simulink model "Project_Observer_Continuous"  (R2014a)
settings: Solver=ode45  StartTime=0.0  StopTime=5  RelTol=1e-3
values from neighbouring files (symbols this model uses):
  A = [-(Kt*Kb/Ra/Je+Be/Je),0;1,0]    [Lab_6_01.m]
  B = [Kt/Ra/Je;0]    [Lab_6_01.m]
  Be = Bm    (= 0.02)    [Lab_6_01.m]
  C = [0,rm*r2/r1]    [Lab_6_01.m]
  Je = Jo+Jm+(rm/r1)^2*(J1+J2)+mc*(rm*r2/r1)^2+J3*(rm*r2/(r1*r3))^2    [Lab_6_01.m]
  K = [0,1]*(Pc^-1)*qa    [Lab_6_01.m]
  Kb = 0.060    (= 0.06)    [Lab_6_01.m]
  Kt = 0.065    [Lab_6_01.m]
  L = pa*Po^-1*[0;1]    [Lab_6_01.m]
  La = 0    [Lab_6_01.m]
  n = rm*r2/r1    (= 0.15)    [Lab_6_01.m]
  pos = input('Enter desired steady-state position [mm]: ')/1000    [Lab_6_01.m]
  Ra = 1.5    [Lab_6_01.m]
  ramp = input('Enter desired steady-state velocity [mm/s]: ')/1000    [Lab_6_01.m]
  Ramp_On = 1    [Lab_6_01.m]
  SampleTime = 0.01    [Lab_6_01.m]
  Step_On = 0    [Lab_6_01.m]
libraries: simulink x1
settings Model: Creator=muellerb  LastModifiedBy=cloughj

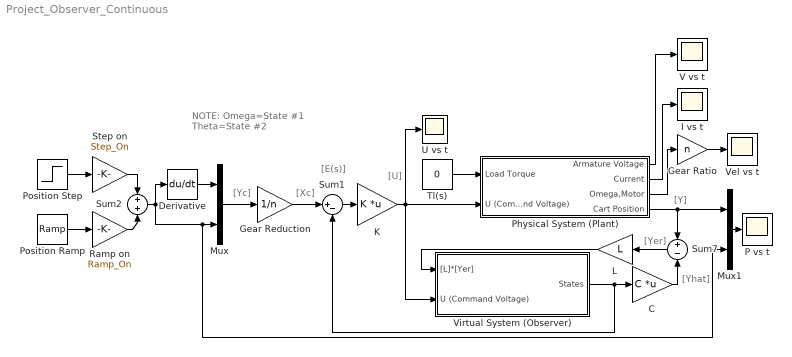
== system Project_Observer_Continuous ==
  note: [Yhat]
  note: [Yer]
  note: [Y]
  note: [U]
  note: [E(s)]
  note: [Xc]
  note: [Yc]
  note: NOTE:
      | Omega=State #1
      | Theta=State #2
  C : Gain  Gain=C  Multiplication=Matrix(K*u)
  Derivative : Derivative
  Gear Ratio : Gain  Gain=n
  Gear Reduction : Gain  Gain=1/n
  I vs t : Scope
      settings: SaveName=Current
  K : Gain  Gain=K  Multiplication=Matrix(K*u)
  L : Gain  Gain=L
  Mux : Mux  Inputs=2
  Mux1 : Mux  Inputs=2
  P vs t : Scope
      settings: SaveName=Position
  Physical System (Plant) : Subsystem
  Position Ramp : simulink/Sources/Ramp  slope=ramp  start=0  X0=0
  Position Step : Step  Time=0  After=pos  SampleTime=SampleTime
  Ramp on : Gain  Gain=Ramp_On
  Step on : Gain  Gain=Step_On
  Sum1 : Sum  Inputs=|+-
  Sum2 : Sum  Inputs=+|+
  Sum7 : Sum  Inputs=+|-
  Tl(s) : Constant  Value=0
  U vs t : Scope
      settings: SaveName=ScopeData4
  V vs t : Scope
      settings: SaveName=Voltage
  Vel vs t : Scope
      settings: SaveName=ScopeData3
  Virtual System (Observer) : Subsystem
  wires:
  Gear Ratio/1 -> Vel vs t/1
  Sum7/1 -> L/1
  Mux/1 -> Gear Reduction/1
  Gear Reduction/1 -> Sum1/1
  Sum1/1 -> K/1
  Tl(s)/1 -> Physical System (Plant)/1(Load Torque)
  Physical System (Plant)/1(Armature Voltage) -> V vs t/1
  Physical System (Plant)/2(Current) -> I vs t/1
  Physical System (Plant)/3(Omega,Motor) -> Gear Ratio/1
  Physical System (Plant)/4(Cart Position) -> Sum7/1, Mux1/1
  L/1 -> Virtual System (Observer)/1("[L]*[Yer]")
  C/1 -> Sum7/2
  Virtual System (Observer)/1(States) -> Sum1/2, C/1
  Position Ramp/1 -> Ramp on/1
  Position Step/1 -> Step on/1
  Step on/1 -> Sum2/1
  Ramp on/1 -> Sum2/2
  K/1 -> U vs t/1, Virtual System (Observer)/2(U (Command Voltage)), Physical System (Plant)/2(U (Command Voltage))
  Derivative/1 -> Mux/1
  Sum2/1 -> Mux1/2, Mux/2, Derivative/1
  Mux1/1 -> P vs t/1

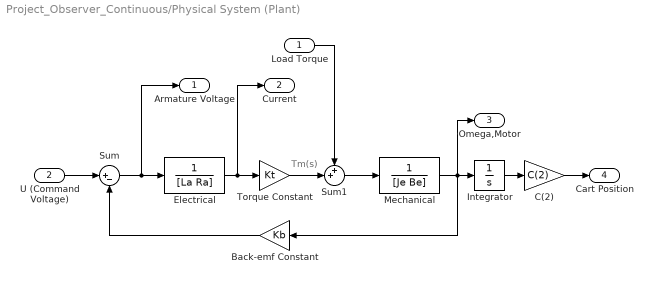
== system Project_Observer_Continuous/Physical System (Plant) ==
  note: Tm(s)
  Load Torque : Inport
  U (Command Voltage) : Inport  Port=2
  Back-emf Constant : Gain  Gain=Kb
  C(2) : Gain  Gain=C(2)
  Electrical : TransferFcn  Denominator=[La Ra]
  Integrator : Integrator
  Mechanical : TransferFcn  Denominator=[Je Be]
  Sum : Sum  Inputs=|+-
  Sum1 : Sum  Inputs=++|
  Torque Constant : Gain  Gain=Kt
  Armature Voltage : Outport
  Current : Outport  Port=2
  Omega,Motor : Outport  Port=3
  Cart Position : Outport  Port=4
  wires:
  Sum/1 -> Armature Voltage/1, Electrical/1
  Electrical/1 -> Current/1, Torque Constant/1
  Sum1/1 -> Mechanical/1
  Back-emf Constant/1 -> Sum/2
  Torque Constant/1 -> Sum1/2
  Load Torque/1 -> Sum1/1
  Mechanical/1 -> Back-emf Constant/1, Omega,Motor/1, Integrator/1
  U (Command Voltage)/1 -> Sum/1
  Integrator/1 -> C(2)/1
  C(2)/1 -> Cart Position/1

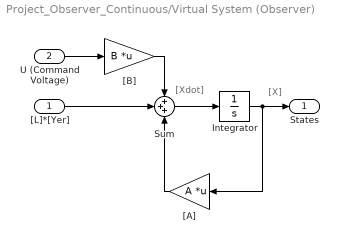
== system Project_Observer_Continuous/Virtual System (Observer) ==
  note: [X]
  note: [Xdot]
  "[L]*[Yer]" : Inport
  U (Command Voltage) : Inport  Port=2
  Integrator : Integrator
  Sum : Sum  Inputs=+++
  "[A]" : Gain  Gain=A  Multiplication=Matrix(K*u)
  "[B]" : Gain  Gain=B  Multiplication=Matrix(K*u)
  States : Outport
  wires:
  U (Command Voltage)/1 -> "[B]"/1
  "[B]"/1 -> Sum/1
  "[L]*[Yer]"/1 -> Sum/2
  "[A]"/1 -> Sum/3
  Integrator/1 -> States/1, "[A]"/1
  Sum/1 -> Integrator/1
